simulink model "QBot2_IMAGE_DOWNSAMPLING"  (Simulink 8.6)
settings: Solver=ode1  StartTime=0.0  StopTime=inf  FixedStep=0.01  RelTol=1e-3
undefined symbols (not defined in the file): HIL, Kinect, qc_get_step_size
libraries: quarc_library x13
settings Model: Creator=drmadill  LastModifiedBy=rclue  SimulationMode=external  ExtModeTrigDuration=1
settings SolverCC: PositivePriorityOrder=on
settings DebuggingCC: FcnCallInpInsideContextMsg=UseLocalSettings
settings RTWCC: SystemTargetFile=quarc_linux_duovero.tlc  TemplateMakefile=quarc_linux_duovero_tmf  Description=QUARC Linux DuoVero Target
settings STFCustomTargetCC: TargetLibSuffix=.a  TargetPreCompLibLocation=C:\PROGRA~3\QUARC\lib\2015b\LINUX_~1\release  ConcurrentExecutionCompliant=on  GeneratePreprocessorConditionals=Disable all  CPPClassGenCompliant=on  SystemTargetFile=quarc_linux_duovero.tlc
settings GRTTargetCC: TargetLibSuffix=.a  TargetPreCompLibLocation=C:\PROGRA~3\QUARC\lib\2015b\LINUX_~1\release  ParMdlRefBuildCompliant=off  CompOptLevelCompliant=off  MatFileLogging=off  UseToolchainInfoCompliant=off  ExtMode=on  ExtModeMexFile=quarc_comm  ExtModeMexArgs='-w -d /tmp -uri %u', 'tcpip://192.168.2.49:17001'

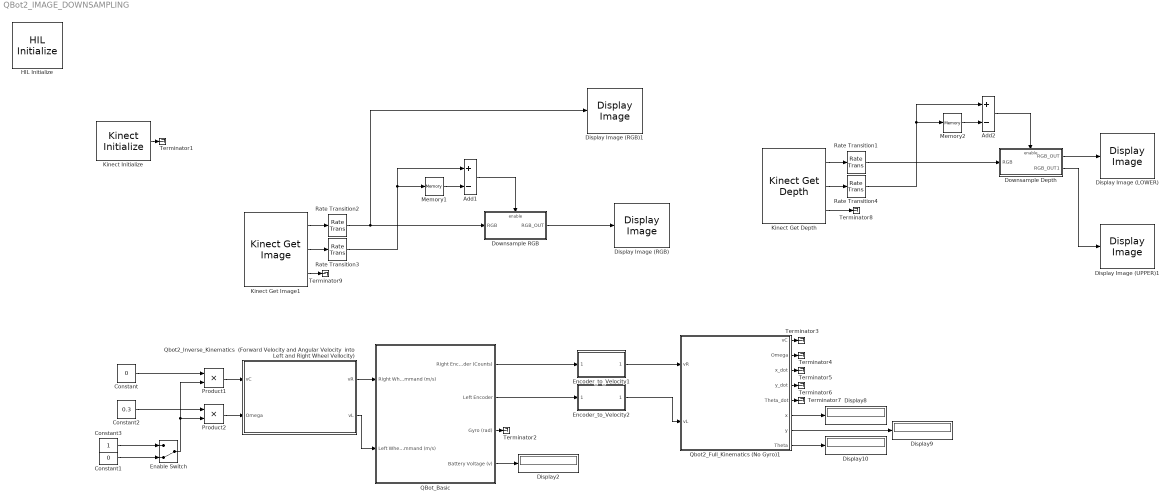
== system QBot2_IMAGE_DOWNSAMPLING ==
  Add1 : Sum  Inputs=+-
  Add2 : Sum  Inputs=+-
  Constant : Constant  Value=0
  Constant1 : Constant  Value=0
  Constant2 : Constant  Value=0.3
  Constant3 : Constant
  Display Image (LOWER) : quarc_library/Sinks/Figures/Display Image  figure_mode=Use figure window  figure_tag=figure1  axes_tag=axes1  update_rate=1  initial_position="39  232  854  629"  initial_visibility=off  sample_time=-1  axes_only=off  orig_size=off
  Display Image (RGB) : quarc_library/Sinks/Figures/Display Image  figure_mode=Use figure window  figure_tag=figure1  axes_tag=axes1  update_rate=1  initial_position="450  265  776  575"  initial_visibility=off  sample_time=-1  axes_only=off  orig_size=off
  Display Image (RGB)1 : quarc_library/Sinks/Figures/Display Image  figure_mode=Use figure window  figure_tag=figure1  axes_tag=axes1  update_rate=1  initial_position="281  313  776  575"  initial_visibility=off  sample_time=-1  axes_only=off  orig_size=off
  Display Image (UPPER)1 : quarc_library/Sinks/Figures/Display Image  figure_mode=Use figure window  figure_tag=figure1  axes_tag=axes1  update_rate=1  initial_position="833  202  808  676"  initial_visibility=off  sample_time=-1  axes_only=off  orig_size=off
  Display{2,8..10} (4 alike) : Display
  Downsample Depth : Subsystem  TreatAsAtomicUnit=on
  Downsample RGB : Subsystem  TreatAsAtomicUnit=on
  Enable Switch : ManualSwitch  CurrentSetting=0
  Encoder_to_Velocity1 : Subsystem
  Encoder_to_Velocity2 : Subsystem
  HIL Initialize : quarc_library/Data Acquisition/Generic/Configuration/HIL Initialize  Priority=-99  object_name=HIL-1  board_type=qbot2  board_number=0  board_options=enc0_dir=0;enc0_filter=1;enc0_a=0;enc0_b=0;enc0_z=1;enc0_reload=0;enc1_dir=0;enc1_filter=1;enc1_a=0;enc1_b=0;enc1_z=1;enc1_reload=0;pwm0_immediate=0;pwm1_immediate=0;pwm2_immediate=0;pwm3_immediate=0;  exclusive=off  active=off  hardware_clocks=[]  clock_modes=[]  initial_clock_frequencies=[]  set_clock_params_at_start=off  set_clock_params_at_switch_in=off  set_clock_frequencies_at_start=off  set_clock_frequencies_at_switch_in=off  analog_input_channels=[0:9]  analog_input_maximums=[5 5 5 5 16.5 3.3 3.3 3.3 3.3]  analog_input_minimums=[0 0 0 0 0 0 0 0 0]  set_analog_input_params_at_start=off  set_analog_input_params_at_switch_in=off  analog_output_channels=[]  analog_output_maximums=[]  analog_output_minimums=[]  initial_analog_outputs=[]  final_analog_outputs=[]  watchdog_analog_outputs=[]  set_analog_output_params_at_start=off  set_analog_output_params_at_switch_in=off  set_analog_outputs_at_start=off  set_analog_outputs_at_switch_in=off  set_analog_outputs_at_terminate=off  set_analog_outputs_at_switch_out=off  set_analog_outputs_on_watchdog=off  digital_input_channels=[]  digital_output_channels=[]  digital_output_configuration=[]  initial_digital_outputs=[0]  final_digital_outputs=[0]  watchdog_digital_outputs=[0]  set_digital_output_params_at_start=off  set_digital_output_params_at_switch_in=off  set_digital_outputs_at_start=on  set_digital_outputs_at_switch_in=off  set_digital_outputs_at_terminate=on  set_digital_outputs_at_switch_out=off  set_digital_outputs_on_watchdog=on  encoder_channels=[0:3]  quadrature=[4]  encoder_filter_frequency=[]  initial_encoder_counts=[0]  set_encoder_params_at_start=on  set_encoder_params_at_switch_in=off  set_encoder_counts_at_start=on  set_encoder_counts_at_switch_in=off  pwm_channels=[0:3]  pwm_modes=[0]  pwm_frequency=[20e6/1024]  pwm_configuration=[0]  pwm_alignment=[0]  pwm_polarity=[1]  pwm_leading_deadband=[0]  pwm_trailing_deadband=[0]  initial_pwm_outputs=[0]  final_pwm_outputs=[0]  watchdog_pwm_outputs=[0]  set_pwm_params_at_start=on  set_pwm_params_at_switch_in=off  set_pwm_outputs_at_start=on  set_pwm_outputs_at_switch_in=off  set_pwm_outputs_at_terminate=on  set_pwm_outputs_at_switch_out=off  set_pwm_outputs_on_watchdog=on  other_output_channels=[2000:2001 14000 16000]  initial_other_outputs=[0 0 0 7]  final_other_outputs=[0 0 0 7]  watchdog_other_outputs=[]  set_other_outputs_at_start=on  set_other_outputs_at_switch_in=off  set_other_outputs_at_terminate=on  set_other_outputs_at_switch_out=off  set_other_outputs_on_watchdog=off
  Kinect Get Depth : quarc_library/Multimedia/Kinect Get Depth  object_name=Kinect-1  resolution=640 x 480  sample_time=qc_get_step_size * ceil(0.033 / qc_get_step_size)  show_player=off
  Kinect Get Image1 : quarc_library/Multimedia/Kinect Get Image  object_name=Kinect-1  sensor_type=color  resolution=640 x 480  output_format=MATLAB RGB (HxWx3)  data_type=uint8  backlight=average brightness  flicker=none  brightness=0.2156  gain=1.0  gamma=2.2  autoexposure=on  exposure=0  contrast=1.0  sharpness=0.5  hue=0.0  saturation=1.0  autobalance=on  balance=2700  frame_interval=0  sample_time=qc_get_step_size * ceil(0.033 / qc_get_step_size)
  Kinect Initialize : quarc_library/Multimedia/Kinect Initialize  object_name=Kinect-1  kinect_type=Kinect for XBox 360  identifier=0  sample_time=qc_get_step_size * ceil(0.033 / qc_get_step_size)  active=on
  Memory1 : Memory
  Memory2 : Memory
  Product1 : Product  RndMeth=Zero
  Product2 : Product  RndMeth=Zero
  QBot_Basic : Subsystem
  Qbot2_Full_Kinematics (No Gyro)1 : Subsystem
  Qbot2_Inverse_Kinematics  (Forward Velocity and Angular Velocity  into Left and Right Wheel Vellocity) : Subsystem
  Rate Transition{1..4} (4 alike) : RateTransition
  Terminator{1..9} (9 alike) : Terminator
  wires:
  Constant3/1 -> Enable Switch/1
  Constant1/1 -> Enable Switch/2
  QBot_Basic/1(Right Encoder (Counts)) -> Encoder_to_Velocity1/1(Encoder)
  QBot_Basic/2(Left Encoder) -> Encoder_to_Velocity2/1(Encoder)
  QBot_Basic/4(Battery Voltage (v)) -> Display2/1
  Qbot2_Full_Kinematics (No Gyro)1/8(Theta) -> Display10/1
  Qbot2_Full_Kinematics (No Gyro)1/7(y) -> Display9/1
  Qbot2_Full_Kinematics (No Gyro)1/6(x) -> Display8/1
  Encoder_to_Velocity1/1(Velocity) -> Qbot2_Full_Kinematics (No Gyro)1/1(vR)
  Encoder_to_Velocity2/1(Velocity) -> Qbot2_Full_Kinematics (No Gyro)1/2(vL)
  Constant/1 -> Product1/1
  Constant2/1 -> Product2/1
  Qbot2_Inverse_Kinematics  (Forward Velocity and Angular Velocity  into Left and Right Wheel Vellocity)/1(vR) -> QBot_Basic/1(Right Wheel Command (m/s))
  Qbot2_Inverse_Kinematics  (Forward Velocity and Angular Velocity  into Left and Right Wheel Vellocity)/2(vL) -> QBot_Basic/2(Left Wheel Command (m/s))
  Product1/1 -> Qbot2_Inverse_Kinematics  (Forward Velocity and Angular Velocity  into Left and Right Wheel Vellocity)/1(vC)
  Product2/1 -> Qbot2_Inverse_Kinematics  (Forward Velocity and Angular Velocity  into Left and Right Wheel Vellocity)/2(Omega)
  Enable Switch/1 -> Product2/2, Product1/2
  Kinect Initialize/1 -> Terminator1/1
  QBot_Basic/3(Gyro (rad)) -> Terminator2/1
  Qbot2_Full_Kinematics (No Gyro)1/1(vC) -> Terminator3/1
  Qbot2_Full_Kinematics (No Gyro)1/2(Omega) -> Terminator4/1
  Qbot2_Full_Kinematics (No Gyro)1/3(x_dot) -> Terminator5/1
  Qbot2_Full_Kinematics (No Gyro)1/4(y_dot) -> Terminator6/1
  Qbot2_Full_Kinematics (No Gyro)1/5(Theta_dot) -> Terminator7/1
  Kinect Get Image1/1 -> Rate Transition2/1
  Kinect Get Image1/2 -> Rate Transition3/1
  Rate Transition3/1 -> Add1/1, Memory1/1
  Memory1/1 -> Add1/2
  Kinect Get Image1/3 -> Terminator9/1
  Add1/1 -> Downsample RGB/Enable
  Rate Transition2/1 -> Display Image (RGB)1/1, Downsample RGB/1(RGB)
  Downsample RGB/1(RGB_OUT) -> Display Image (RGB)/1
  Rate Transition4/1 -> Add2/1, Memory2/1
  Memory2/1 -> Add2/2
  Kinect Get Depth/1 -> Rate Transition1/1
  Kinect Get Depth/2 -> Rate Transition4/1
  Kinect Get Depth/3 -> Terminator8/1
  Rate Transition1/1 -> Downsample Depth/1(RGB)
  Add2/1 -> Downsample Depth/Enable
  Downsample Depth/1(RGB_OUT) -> Display Image (LOWER)/1
  Downsample Depth/2(RGB_OUT1) -> Display Image (UPPER)1/1

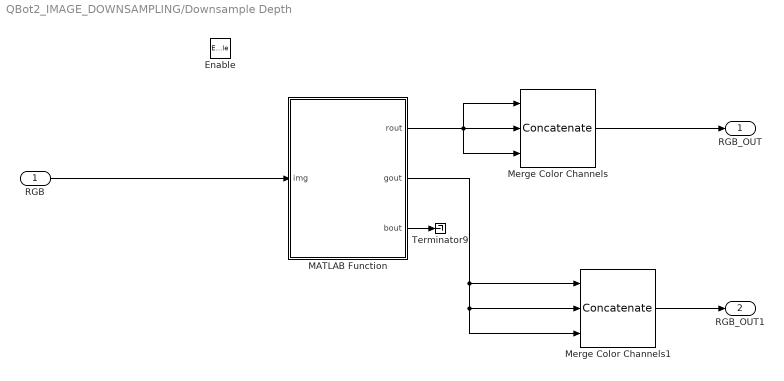
== system QBot2_IMAGE_DOWNSAMPLING/Downsample Depth ==
  RGB : Inport
  Enable : EnablePort
  MATLAB Function : MATLAB Function  TreatAsAtomicUnit=on
  Merge Color Channels : Concatenate  NumInputs=3  Mode=Multidimensional array  ConcatenateDimension=3
  Merge Color Channels1 : Concatenate  NumInputs=3  Mode=Multidimensional array  ConcatenateDimension=3
  Terminator9 : Terminator
  RGB_OUT : Outport
  RGB_OUT1 : Outport  Port=2
  wires:
  RGB/1 -> MATLAB Function/1(img)
  MATLAB Function/1(rout) -> Merge Color Channels/3, Merge Color Channels/2, Merge Color Channels/1
  Merge Color Channels/1 -> RGB_OUT/1
  Merge Color Channels1/1 -> RGB_OUT1/1
  MATLAB Function/2(gout) -> Merge Color Channels1/3, Merge Color Channels1/2, Merge Color Channels1/1
  MATLAB Function/3(bout) -> Terminator9/1

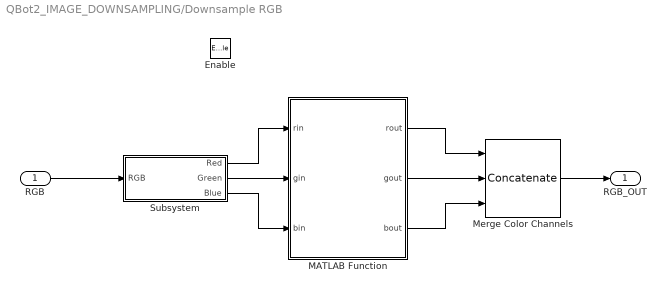
== system QBot2_IMAGE_DOWNSAMPLING/Downsample RGB ==
  RGB : Inport
  Enable : EnablePort
  MATLAB Function : MATLAB Function  TreatAsAtomicUnit=on
  Merge Color Channels : Concatenate  NumInputs=3  Mode=Multidimensional array  ConcatenateDimension=3
  Subsystem : Subsystem
  RGB_OUT : Outport
  wires:
  RGB/1 -> Subsystem/1(RGB)
  Subsystem/2(Green) -> MATLAB Function/2(gin)
  Subsystem/1(Red) -> MATLAB Function/1(rin)
  Subsystem/3(Blue) -> MATLAB Function/3(bin)
  MATLAB Function/1(rout) -> Merge Color Channels/1
  MATLAB Function/2(gout) -> Merge Color Channels/2
  MATLAB Function/3(bout) -> Merge Color Channels/3
  Merge Color Channels/1 -> RGB_OUT/1

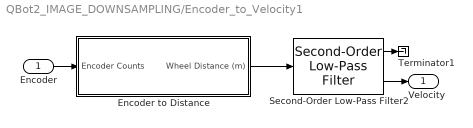
== system QBot2_IMAGE_DOWNSAMPLING/Encoder_to_Velocity1 ==
  Encoder : Inport
  Encoder to Distance : Subsystem
  Second-Order Low-Pass Filter2 : quarc_library/Continuous/Second-Order Low-Pass Filter  params_source=Internal (dialog parameters)  input_width=10  input_zeta=1  input_init=0
  Terminator1 : Terminator
  Velocity : Outport
  wires:
  Second-Order Low-Pass Filter2/2 -> Velocity/1
  Encoder/1 -> Encoder to Distance/1(Encoder Counts)
  Encoder to Distance/1(Wheel Distance (m)) -> Second-Order Low-Pass Filter2/1
  Second-Order Low-Pass Filter2/1 -> Terminator1/1

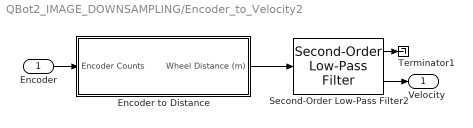
== system QBot2_IMAGE_DOWNSAMPLING/Encoder_to_Velocity2 ==
  Encoder : Inport
  Encoder to Distance : Subsystem
  Second-Order Low-Pass Filter2 : quarc_library/Continuous/Second-Order Low-Pass Filter  params_source=Internal (dialog parameters)  input_width=10  input_zeta=1  input_init=0
  Terminator1 : Terminator
  Velocity : Outport
  wires:
  Second-Order Low-Pass Filter2/1 -> Terminator1/1
  Encoder to Distance/1(Wheel Distance (m)) -> Second-Order Low-Pass Filter2/1
  Encoder/1 -> Encoder to Distance/1(Encoder Counts)
  Second-Order Low-Pass Filter2/2 -> Velocity/1

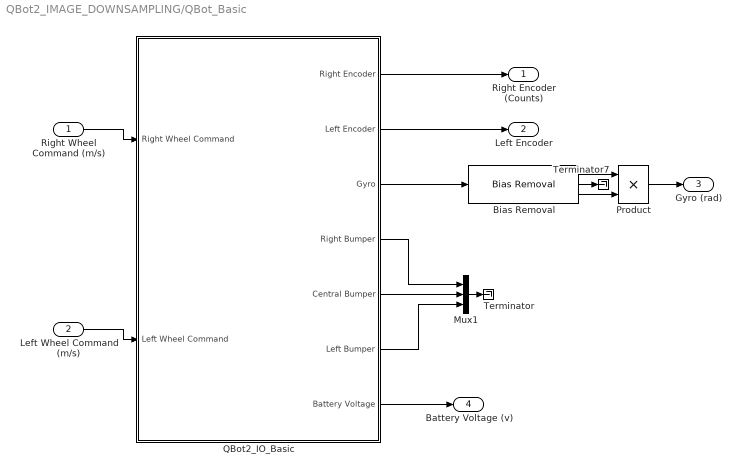
== system QBot2_IMAGE_DOWNSAMPLING/QBot_Basic ==
  Right Wheel Command (m/s) : Inport
  Left Wheel Command (m/s) : Inport  Port=2
  Bias Removal : quarc_library/Discrete/Bias Removal  start_time=3  end_time=4  switch_id=0  sample_time=qc_get_step_size
  Mux1 : Mux  Inputs=3
  Product : Product  RndMeth=Zero
  QBot2_IO_Basic : Subsystem
  Terminator : Terminator
  Terminator7 : Terminator
  Right Encoder (Counts) : Outport
  Left Encoder : Outport  Port=2
  Gyro (rad) : Outport  Port=3
  Battery Voltage (v) : Outport  Port=4
  wires:
  Mux1/1 -> Terminator/1
  QBot2_IO_Basic/3(Gyro) -> Bias Removal/1
  Product/1 -> Gyro (rad)/1
  Bias Removal/3 -> Product/2
  Bias Removal/1 -> Product/1
  Bias Removal/2 -> Terminator7/1
  QBot2_IO_Basic/7(Battery Voltage) -> Battery Voltage (v)/1
  QBot2_IO_Basic/2(Left Encoder) -> Left Encoder/1
  QBot2_IO_Basic/1(Right Encoder) -> Right Encoder (Counts)/1
  Left Wheel Command (m/s)/1 -> QBot2_IO_Basic/2(Left Wheel Command)
  Right Wheel Command (m/s)/1 -> QBot2_IO_Basic/1(Right Wheel Command)
  QBot2_IO_Basic/6(Left Bumper) -> Mux1/3
  QBot2_IO_Basic/5(Central Bumper) -> Mux1/2
  QBot2_IO_Basic/4(Right Bumper) -> Mux1/1

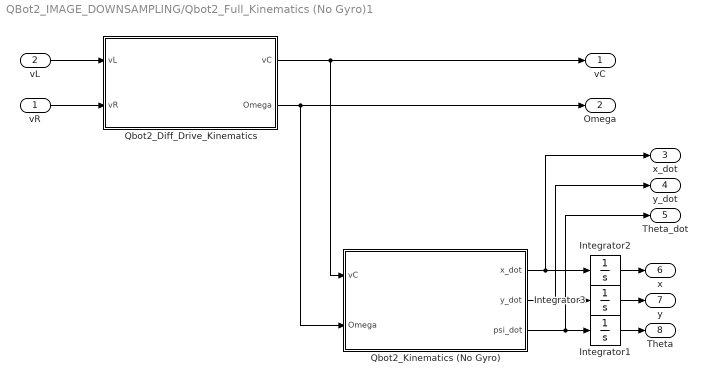
== system QBot2_IMAGE_DOWNSAMPLING/Qbot2_Full_Kinematics (No Gyro)1 ==
  vR : Inport
  vL : Inport  Port=2
  Integrator1 : Integrator
  Integrator2 : Integrator
  Integrator3 : Integrator
  Qbot2_Diff_Drive_Kinematics : Subsystem
  Qbot2_Kinematics (No Gyro) : Subsystem
  vC : Outport
  Omega : Outport  Port=2
  x_dot : Outport  Port=3
  y_dot : Outport  Port=4
  Theta_dot : Outport  Port=5
  x : Outport  Port=6
  y : Outport  Port=7
  Theta : Outport  Port=8
  wires:
  Qbot2_Diff_Drive_Kinematics/2(Omega) -> Omega/1, Qbot2_Kinematics (No Gyro)/2(Omega)
  Integrator3/1 -> y/1
  Integrator2/1 -> x/1
  vR/1 -> Qbot2_Diff_Drive_Kinematics/2(vR)
  vL/1 -> Qbot2_Diff_Drive_Kinematics/1(vL)
  Qbot2_Diff_Drive_Kinematics/1(vC) -> vC/1, Qbot2_Kinematics (No Gyro)/1(vC)
  Qbot2_Kinematics (No Gyro)/2(y_dot) -> Integrator3/1, y_dot/1
  Qbot2_Kinematics (No Gyro)/1(x_dot) -> Integrator2/1, x_dot/1
  Qbot2_Kinematics (No Gyro)/3(psi_dot) -> Integrator1/1, Theta_dot/1
  Integrator1/1 -> Theta/1

== system QBot2_IMAGE_DOWNSAMPLING/Qbot2_Inverse_Kinematics  (Forward Velocity and Angular Velocity  into Left and Right Wheel Vellocity) ==
  vC : Inport
  Omega : Inport  Port=2
  Qbot2_Inverse_Kinematics  (Forward Velocity and Angular Velocity into Left and Right Wheel Vellocity) : MATLAB Function  TreatAsAtomicUnit=on
  vR : Outport
  vL : Outport  Port=2
  wires:
  vC/1 -> Qbot2_Inverse_Kinematics  (Forward Velocity and Angular Velocity into Left and Right Wheel Vellocity)/1(vC)
  Qbot2_Inverse_Kinematics  (Forward Velocity and Angular Velocity into Left and Right Wheel Vellocity)/1(vR) -> vR/1
  Omega/1 -> Qbot2_Inverse_Kinematics  (Forward Velocity and Angular Velocity into Left and Right Wheel Vellocity)/2(Omega)
  Qbot2_Inverse_Kinematics  (Forward Velocity and Angular Velocity into Left and Right Wheel Vellocity)/2(vL) -> vL/1

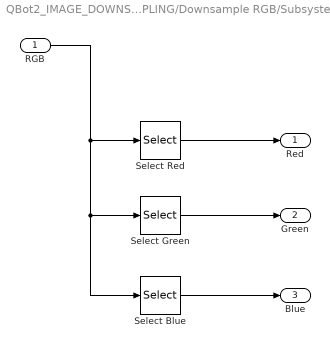
== system QBot2_IMAGE_DOWNSAMPLING/Downsample RGB/Subsystem ==
  RGB : Inport
  Select Blue : Selector  NumberOfDimensions=3  InputPortWidth=3  IndexOptions=Select all,Select all,Index vector (dialog)  Indices=[1 3],1,3  OutputSizes=1,1,1
  Select Green : Selector  NumberOfDimensions=3  InputPortWidth=3  IndexOptions=Select all,Select all,Index vector (dialog)  Indices=[1 3],1,2  OutputSizes=1,1,1
  Select Red : Selector  NumberOfDimensions=3  InputPortWidth=3  IndexOptions=Select all,Select all,Index vector (dialog)  Indices=[1 3],1,1  OutputSizes=1,1,1
  Red : Outport
  Green : Outport  Port=2
  Blue : Outport  Port=3
  wires:
  Select Red/1 -> Red/1
  Select Green/1 -> Green/1
  Select Blue/1 -> Blue/1
  RGB/1 -> Select Blue/1, Select Green/1, Select Red/1

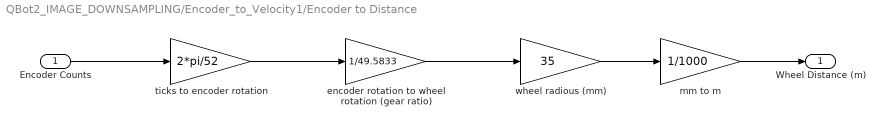
== system QBot2_IMAGE_DOWNSAMPLING/Encoder_to_Velocity1/Encoder to Distance ==
  Encoder Counts : Inport
  " encoder rotation to wheel rotation (gear ratio)" : Gain  Gain=1/49.5833
  mm to m : Gain  Gain=1/1000
  ticks to encoder rotation : Gain  Gain=2*pi/52
  wheel radious (mm) : Gain  Gain=35
  Wheel Distance (m) : Outport
  wires:
  mm to m/1 -> Wheel Distance (m)/1
  wheel radious (mm)/1 -> mm to m/1
  " encoder rotation to wheel rotation (gear ratio)"/1 -> wheel radious (mm)/1
  ticks to encoder rotation/1 -> " encoder rotation to wheel rotation (gear ratio)"/1
  Encoder Counts/1 -> ticks to encoder rotation/1

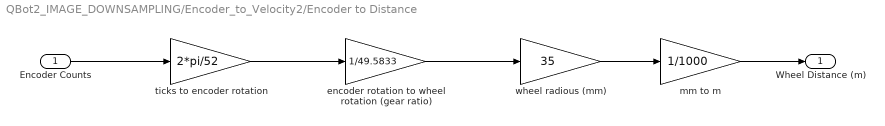
== system QBot2_IMAGE_DOWNSAMPLING/Encoder_to_Velocity2/Encoder to Distance ==
  Encoder Counts : Inport
  " encoder rotation to wheel rotation (gear ratio)" : Gain  Gain=1/49.5833
  mm to m : Gain  Gain=1/1000
  ticks to encoder rotation : Gain  Gain=2*pi/52
  wheel radious (mm) : Gain  Gain=35
  Wheel Distance (m) : Outport
  wires:
  Encoder Counts/1 -> ticks to encoder rotation/1
  ticks to encoder rotation/1 -> " encoder rotation to wheel rotation (gear ratio)"/1
  " encoder rotation to wheel rotation (gear ratio)"/1 -> wheel radious (mm)/1
  wheel radious (mm)/1 -> mm to m/1
  mm to m/1 -> Wheel Distance (m)/1

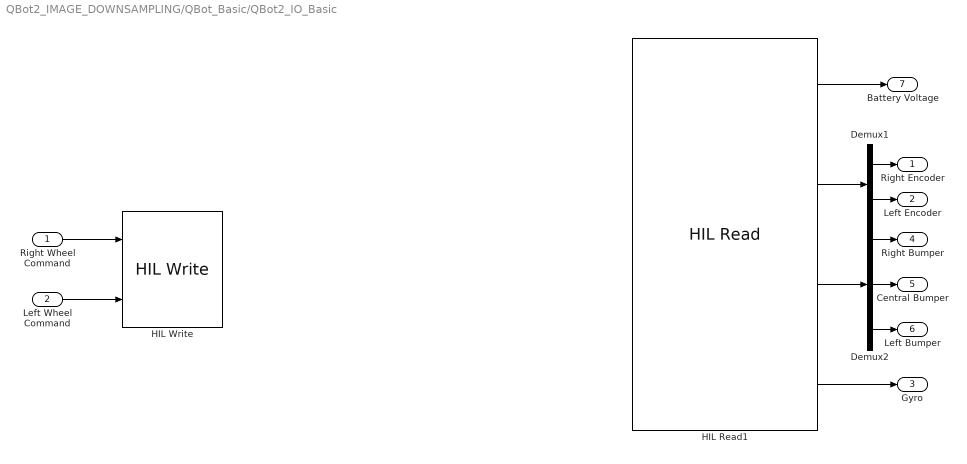
== system QBot2_IMAGE_DOWNSAMPLING/QBot_Basic/QBot2_IO_Basic ==
  Right Wheel Command : Inport
  Left Wheel Command : Inport  Port=2
  Demux1 : Demux  Outputs=2
  Demux2 : Demux  Outputs=3
  HIL Read1 : quarc_library/Data Acquisition/Generic/Immediate I//O/HIL Read  object_name=HIL-1  analog_channels=[4]  encoder_channels=[2 3]  digital_channels=[8 9 10]  other_channels=[1002]  sample_time=qc_get_step_size  active=on  vector_output=on  data_type_mode=Inherit via back propagation  encoder_data_type=double  digital_data_type=boolean
  HIL Write : quarc_library/Data Acquisition/Generic/Immediate I//O/HIL Write  object_name=HIL-1  analog_channels=[]  pwm_channels=[]  digital_channels=[]  other_channels=[2000:2001]  sample_time=-1  active=on  vector_input=off
  Right Encoder : Outport
  Left Encoder : Outport  Port=2
  Gyro : Outport  Port=3
  Right Bumper : Outport  Port=4
  Central Bumper : Outport  Port=5
  Left Bumper : Outport  Port=6
  Battery Voltage : Outport  Port=7
  wires:
  Demux2/3 -> Left Bumper/1
  Demux2/2 -> Central Bumper/1
  Demux2/1 -> Right Bumper/1
  HIL Read1/2 -> Demux1/1
  Left Wheel Command/1 -> HIL Write/2
  Right Wheel Command/1 -> HIL Write/1
  Demux1/2 -> Left Encoder/1
  Demux1/1 -> Right Encoder/1
  HIL Read1/4 -> Gyro/1
  HIL Read1/3 -> Demux2/1
  HIL Read1/1 -> Battery Voltage/1

== system QBot2_IMAGE_DOWNSAMPLING/Qbot2_Full_Kinematics (No Gyro)1/Qbot2_Diff_Drive_Kinematics ==
  vL : Inport
  vR : Inport  Port=2
  Qbot2_Diff_Drive_Kinematics : MATLAB Function  TreatAsAtomicUnit=on
  vC : Outport
  Omega : Outport  Port=2
  wires:
  Qbot2_Diff_Drive_Kinematics/2(Omega) -> Omega/1
  vR/1 -> Qbot2_Diff_Drive_Kinematics/2(vR)
  Qbot2_Diff_Drive_Kinematics/1(vC) -> vC/1
  vL/1 -> Qbot2_Diff_Drive_Kinematics/1(vL)

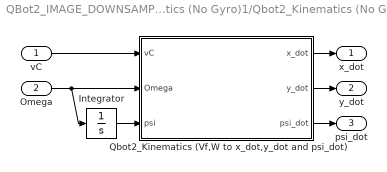
== system QBot2_IMAGE_DOWNSAMPLING/Qbot2_Full_Kinematics (No Gyro)1/Qbot2_Kinematics (No Gyro) ==
  vC : Inport
  Omega : Inport  Port=2
  Integrator : Integrator
  Qbot2_Kinematics (Vf,W to x_dot,y_dot and psi_dot) : MATLAB Function  TreatAsAtomicUnit=on
  x_dot : Outport
  y_dot : Outport  Port=2
  psi_dot : Outport  Port=3
  wires:
  Qbot2_Kinematics (Vf,W to x_dot,y_dot and psi_dot)/2(y_dot) -> y_dot/1
  Omega/1 -> Qbot2_Kinematics (Vf,W to x_dot,y_dot and psi_dot)/2(Omega), Integrator/1
  Qbot2_Kinematics (Vf,W to x_dot,y_dot and psi_dot)/1(x_dot) -> x_dot/1
  vC/1 -> Qbot2_Kinematics (Vf,W to x_dot,y_dot and psi_dot)/1(vC)
  Integrator/1 -> Qbot2_Kinematics (Vf,W to x_dot,y_dot and psi_dot)/3(psi)
  Qbot2_Kinematics (Vf,W to x_dot,y_dot and psi_dot)/3(psi_dot) -> psi_dot/1

== matlab function Downsample Depth/MATLAB Function ==
  data: img input double; rout output double; gout output double; bout output double
function [rout, gout, bout]  = downsample(img)
%#codegen

%constant

rate = 8;
offset = rate/2;
new_row = 60;
new_col = 80;


rout = uint8(zeros(new_row, new_col));
gout = uint8(zeros(new_row, new_col));
bout = uint8(zeros(new_row, new_col));

u = offset;
v = offset;
for i=1:new_row
    for j=1:new_col

        rout(i,j) = uint8(mod(img(u,v), 256));
        gout(i,j) = uint8(bitshift(img(u,v), -8));
        bout(i,j) = uint8(0);
        
        v = v + rate;
    end
    
    v = offset;
    u = u + rate;
end

== matlab function Qbot2_Full_Kinematics (No Gyro)1/Qbot2_Diff_Drive_Kinematics/Qbot2_Diff_Drive_Kinematics ==
  data: vL input double; vC output double; vR input double; Omega output double
function [vC,Omega] = fcn(vL,vR)
%#codegen

d= 0.235;

vC=0.5*(vL+vR);
Omega=(1/d)*(vR-vL);

== matlab function Qbot2_Full_Kinematics (No Gyro)1/Qbot2_Kinematics (No Gyro)/Qbot2_Kinematics (Vf,W to x_dot,y_dot and psi_dot) ==
  data: vC input double; x_dot output double; Omega input double; y_dot output double; psi input double; psi_dot output double
function [x_dot,y_dot,psi_dot] = fcn(vC,Omega,psi)
%#codegen


x_dot=cos(psi)*vC;
y_dot=sin(psi)*vC;
psi_dot= Omega;

== matlab function Downsample RGB/MATLAB Function ==
  data: rin input double; rout output double; gin input double; bin input double; gout output double; bout output double
function [rout, gout, bout] = downsample(rin, gin, bin)
%#codegen

%constant

rate = 8;
offset = rate/2;
new_row = 60;
new_col = 80;

rout = uint8(zeros(new_row,new_col));
gout = uint8(zeros(new_row,new_col));
bout = uint8(zeros(new_row,new_col));


u = offset;
v = offset;
for i=1:new_row
    for j=1:new_col
        
        rout(i,j) = uint8(rin(u,v));
        gout(i,j) = uint8(gin(u,v));
        bout(i,j) = uint8(bin(u,v));
        
        v = v + rate;
    end
    
    v = offset;
    u = u + rate;
end

== matlab function Qbot2_Inverse_Kinematics (Forward Velocity and Angular Velocity into Left and Right Wheel Vellocity)/Qbot2_Inverse_Kinematics (Forward Velocity and Angular Velocity into Left and Right Wheel Vellocity) ==
  data: vR output double; vL output double; vC input double; Omega input double
function [vR,vL] = fcn(vC , Omega)
%#codegen

d=0.235; 
% Eqn Based on the eqn 4.52 (W is the angular velocity)

vR = vC + Omega*d/2;
vL= vC - Omega*d/2;
